simulink model "Quadrotor_Controller"  (R2018b)
settings: Solver=ode14x  StartTime=0.0  StopTime=10  FixedStep=1/100  RelTol=1e-3  EnableMultiTasking=on
undefined symbols (not defined in the file): Ap, cd, DiscIntNeverNeededParam, kt, L, Newton, Pitch_0, Raphson, rho, Roll_0, Rp, X, Y, Z
libraries: sm_lib x122, fl_lib x69, nesl_utility x14, sharedtransform x12, simulink x5, Electrical_Library x4, Mechanical_Library x4
(part 1 of 4)
settings Model: Creator=ppreethi  LastModifiedBy=standard
settings SolverCC: ExtrapolationOrder=2
settings DataIOCC: LimitDataPoints=on  SaveFormat=Array  InspectSignalLogs=on
settings OptimizationCC: BlockReduction=off  DefaultParameterBehavior=Inlined  OptimizeBlockIOStorage=off  BufferReuse=off  GlobalBufferReuse=off  ExpressionFolding=off  LocalBlockOutputs=off  LifeSpan=inf  OptimizeDataStoreBuffers=off  BusAssignmentInplaceUpdate=off
settings DebuggingCC: UnderspecifiedInitializationDetection=Classic  MergeDetectMultiDrivingBlocksExec=none  SolverPrmCheckMsg=warning  ParameterPrecisionLossMsg=none  BusObjectLabelMismatch=error  StateNameClashWarn=warning  StrictBusMsg=ErrorOnBusTreatedAsVector  NonBusSignalsTreatedAsBus=warning  SFUnexpectedBacktrackingDiag=warning  SFNoUnconditionalDefaultTransitionDiag=warning  SFExecutionAtInitializationDiag=none
settings HardwareCC: ProdBitPerPointer=32  ProdBitPerSizeT=32  ProdBitPerPtrDiffT=32  ProdLargestAtomicFloat=None  ProdWordSize=32  ProdHWDeviceType=Generic->32-bit x86 compatible
settings ModelReferenceCC: PropagateSignalLabelsOutOfModel=off
settings SFSimCC: SimUseLocalCustomCode=off
settings RTWCC: SystemTargetFile=xpctarget.tlc  TLCOptions=-axPCModelStackSizeKB=1024  TemplateMakefile=xpc_default_tmf  Description=xPC Target  RTWUseLocalCustomCode=off  RTWCompilerOptimization=on
settings CodeAppCC: StateflowObjectComments=on
settings TargetCC: CodeReplacementLibrary=XPC_BLAS  ParMdlRefBuildCompliant=on  ConcurrentExecutionCompliant=on  MatFileLogging=on  PreserveStateflowLocalDataDimensions=off  MATLABClassNameForMDSCustomization=xpcAperiodicCustomization
settings ConfigComp: CovMetricSettings=dw  CovHtmlReporting=on  CovSaveCumulativeToWorkspaceVar=on  CovSaveSingleToWorkspaceVar=on  CovExternalEMLEnable=off  CovSFcnEnable=off
settings SimscapeCC: SimscapeNormalizeSystem=off
settings ConfigurationSet: Description=SimMechanics 2G
settings ExplorerConfigSet: InternalSimMechanicsExplorerSettings="<ExplorerConfiguration><canonicalview>default</canonicalview><AnimationSetting><BasePlaybackSpeed>1.0</BasePlaybackSpeed><PlaybackSpeedFactor>1.0</PlaybackSpeedFactor></AnimationSetting><TilePanel><TileInfo><Tiles Columns=\"1\" Count=\"1\" Rows=\"1\"><Column Left=\"2\" Weight=\"1\"/><Column Left=\"1669\"/><Row Top=\"2\" Weight=\"1\"/><Row Top=\"1032\"/><Tile Height=\"1\" Width=\"1\" X=\"0\" Y=\"0\"/></Tiles></TileInfo><SceneInfo><SceneViewer><BGColor><R>1</R><G>1</G><B>1</B></BGColor><Camera><Position><X>-0.98734234069472837</X><Y>-2.5766196877608176</Y><Z>-0.21434917441758128</Z></Position><Center><X>-0.36548137966941641</X><Y>0.086653013342029503</Y><Z>0.52407155472837563</Z></Center><Up><X>-0.18648657026384141</X><Y>0.30268994651916503</Y><Z>-0.93466654769893953</Z></Up><Left>-0.88113891027964153</Left><Right>0.88113891027964153</Right><Bottom>-0.94141860281001366</Bottom><Top>0.94141860281001366</Top></Camera></SceneViewer></SceneInfo></TilePanel></ExplorerConfiguration>"

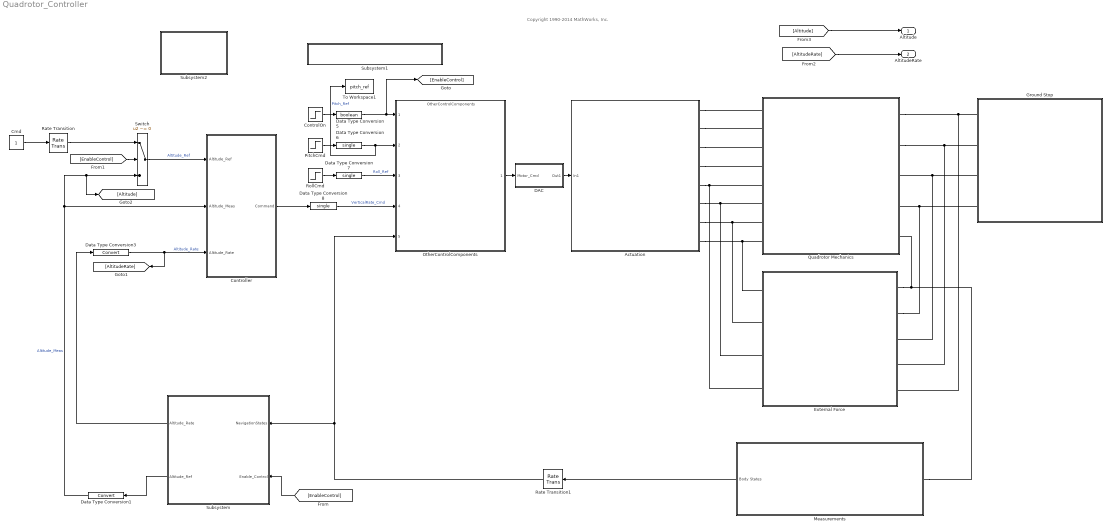
== system Quadrotor_Controller ==
  note: Copyright 1990-2014 MathWorks, Inc.
  Actuation : Subsystem
      mask Display: image('motor.png')
  Cmd : Constant
  ControlOn : Step  Time=5  SampleTime=0.01
  Controller : Subsystem  VariantControl=DesktopMode
  DAC : Subsystem
      mask Display: disp('DAC')
  Data Type Conversion1 : DataTypeConversion
  Data Type Conversion3 : DataTypeConversion
  Data Type Conversion5 : DataTypeConversion  OutDataTypeStr=boolean
  Data Type Conversion6 : DataTypeConversion  OutDataTypeStr=single
  Data Type Conversion7 : DataTypeConversion  OutDataTypeStr=single
  Data Type Conversion8 : DataTypeConversion  OutDataTypeStr=single
  External Force : Subsystem
      mask Display: image('rotor.png')
  Ground Stop : Subsystem  mask{Roll0=Roll_0, Pitch0=Pitch_0, Yaw0=0, Damp=0.7, Spring=1e2, Length=-0.083057999999999979068, GRoll=0, GPitch=0, Alt=1}
      mask prompts: Roll0 "Init Roll"; Pitch0 "Init Pitch"; Yaw0 "Init Yaw"; Damp "Damping"; Spring "Spring Constant"; Length "Distance from Center to Motor"; GRoll "Ground Roll"; GPitch "Ground Pitch"; Alt "Initial Altitude"
      mask init:
      | blk = gcb;
      | if Alt<0
      |     Alt = 0;
      |     set_param(blk,'Alt','0')
      |     warning('Cannot Initialize Below Zero Altitude');
      | end
      mask Display: image('earth.png')
  Measurements : Subsystem
  OtherControlComponents : ModelReference  ModelNameDialog=OtherControlComponents  SimulationMode=Normal  ModelReferenceVersion=1.148
  PitchCmd : Step  Time=8  After=0  SampleTime=0.01
  Quadrotor Mechanics : Subsystem
  Rate Transition : RateTransition  OutPortSampleTime=0.01
  Rate Transition1 : RateTransition
  RollCmd : Step  Time=8  After=0  SampleTime=0.01
  Subsystem : Subsystem
  Subsystem1 : Subsystem
      settings: OpenFcn=|
      | %%Set Variant to Real-time
      | HIL=1;
      | Desktop=0;
      | set_param(gcs,'SimulationMode','external');
      mask Display: disp('Real-time Settings')
  Subsystem2 : Subsystem
      settings: OpenFcn=|
      | %%Set Variant to Real-time
      | HIL=0;
      | Desktop=1;
      | set_param(gcs,'SimulationMode','normal');
      mask Display: disp('Desktop Settings')
  Switch : Switch  Criteria=u2 ~= 0
  To Workspace1 : ToWorkspace  VariableName=pitch_ref  SaveFormat=Timeseries  SampleTime=-1
  Altitude : Outport
  AltitudeRate : Outport  Port=2
  wires:
  Measurements/1(Body States) -> Rate Transition1/1
  PitchCmd/1 -> Data Type Conversion6/1
  RollCmd/1 -> Data Type Conversion7/1
  Rate Transition1/1 -> Subsystem/1(NavigationStates), OtherControlComponents/5
  Subsystem/2(Altitude_Ref) -> Data Type Conversion1/1
  Controller/1(Command) -> Data Type Conversion8/1
  Data Type Conversion1/1 -> Controller/2(Altitude_Meas), Switch/3, [Altitude]  "Altitude_Meas"
  Switch/1 -> Controller/1(Altitude_Ref)  "Altitude_Ref"
  ControlOn/1 -> Data Type Conversion5/1
  Cmd/1 -> Rate Transition/1
  Rate Transition/1 -> Switch/1
  Subsystem/1(Altitude_Rate) -> Data Type Conversion3/1
  Data Type Conversion3/1 -> [AltitudeRate], Controller/3(Altitude_Rate)  "Altitude_Rate"
  [EnableControl] -> Subsystem/2(Enable_Control)
  [EnableControl] -> Switch/2
  Data Type Conversion5/1 -> [EnableControl], OtherControlComponents/1
  Data Type Conversion6/1 -> To Workspace1/1, OtherControlComponents/2  "Pitch_Ref"
  Data Type Conversion7/1 -> OtherControlComponents/3  "Roll_Ref"
  Data Type Conversion8/1 -> OtherControlComponents/4  "VerticalRate_Cmd"
  OtherControlComponents/1 -> DAC/1(Motor_Cmd)
  DAC/1(Out1) -> Actuation/1(In1)
  [Altitude] -> Altitude/1
  [AltitudeRate] -> AltitudeRate/1
  connections:
  Quadrotor Mechanics/LConn8 -- External Force/LConn1 -- Actuation/RConn8
  External Force/LConn2 -- Actuation/RConn7 -- Quadrotor Mechanics/LConn7
  External Force/LConn4 -- Quadrotor Mechanics/LConn5 -- Actuation/RConn5
  Ground Stop/RConn1 -- Quadrotor Mechanics/RConn1 -- External Force/RConn5
  Ground Stop/RConn3 -- External Force/RConn3 -- Quadrotor Mechanics/RConn3
  Ground Stop/RConn2 -- Quadrotor Mechanics/RConn2 -- External Force/RConn4
  Ground Stop/RConn4 -- External Force/RConn2 -- Quadrotor Mechanics/RConn4
  Actuation/RConn4 -- Quadrotor Mechanics/LConn4
  Actuation/RConn3 -- Quadrotor Mechanics/LConn3
  Actuation/RConn2 -- Quadrotor Mechanics/LConn2
  External Force/RConn1 -- Quadrotor Mechanics/RConn5 -- Measurements/LConn1
  Actuation/RConn1 -- Quadrotor Mechanics/LConn1
  Quadrotor Mechanics/LConn6 -- Actuation/RConn6 -- External Force/LConn3

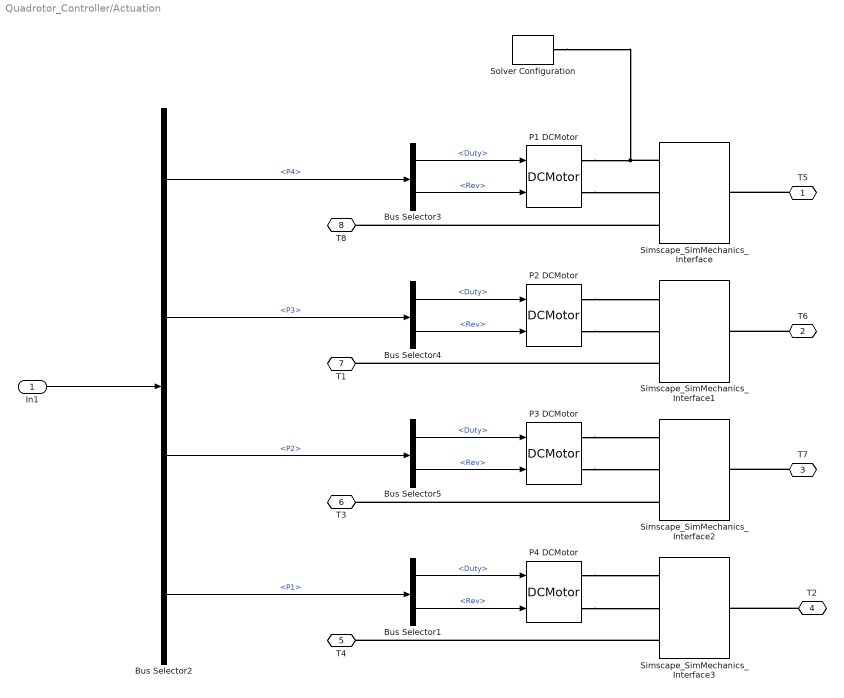
== system Quadrotor_Controller/Actuation ==
  In1 : Inport  OutDataTypeStr=Bus: MotorCommands
  " P1 DCMotor" : Electrical_Library/ DCMotor  SystemSampleTime=-1
  " P2 DCMotor" : Electrical_Library/ DCMotor  SystemSampleTime=-1
  " P3 DCMotor" : Electrical_Library/ DCMotor  SystemSampleTime=-1
  " P4 DCMotor" : Electrical_Library/ DCMotor  SystemSampleTime=-1
  Bus Selector{1,3..5} (4 alike) : BusSelector  OutputSignals=Duty,Rev
  Bus Selector2 : BusSelector  OutputSignals=P4,P3,P2,P1
  Simscape_SimMechanics_Interface{,1..3} (4 alike) : Mechanical_Library/Simscape_SimMechanics_Interface  SystemSampleTime=-1
  Solver Configuration : nesl_utility/Solver Configuration  PhysicalDomain=network_engine_domain  SubClassName=solver  LeftPortType=input  RightPortType=generic  Tones=[]  Harmonics=[]  SimulateNoise=off  Profile=off  UseLocalSampling=off  EnableSwitchedLinearOptims=on  FrequencyDomain=off  UseCCode=off  RelTol=0.001  AbsTol=1e-06  MinStep=1e-09  ToWorkspace=off  RevertToSquareIcSolve=off  NumHomotopyIterations=100  PhasorMode=off  PhasorModeNumHarmonics=1  DoDC=off  ResidualTolerance=1e-09  UseLocalSolver=off  LocalSolverChoice=NE_BACKWARD_EULER_ADVANCER  LocalSolverSampleTime=0.001  DoFixedCost=off  MaxNonlinIter=3  MaxModeIter=2  LinearAlgebra=Sparse  EquationFormulation=NE_TIME_EF  DelaysMemoryBudget=1024  AutomaticFiltering=on  FilteringTimeConstant=0.001  PartitionStorageMethod=AS_NEEDED  PartitionMemoryBudget=1024
  T5 : PMIOPort  Side=Right
  T6 : PMIOPort  Port=2  Side=Right
  T7 : PMIOPort  Port=3  Side=Right
  T2 : PMIOPort  Port=4  Side=Right
  T4 : PMIOPort  Port=5  Side=Right
  T3 : PMIOPort  Port=6  Side=Right
  T1 : PMIOPort  Port=7  Side=Right
  T8 : PMIOPort  Port=8  Side=Right
  wires:
  Bus Selector3/2 -> " P1 DCMotor"/2  "<Rev>"
  Bus Selector3/1 -> " P1 DCMotor"/1  "<Duty>"
  Bus Selector2/1 -> Bus Selector3/1  "<P4>"
  Bus Selector2/4 -> Bus Selector1/1  "<P1>"
  Bus Selector2/2 -> Bus Selector4/1  "<P3>"
  Bus Selector4/2 -> " P2 DCMotor"/2  "<Rev>"
  Bus Selector4/1 -> " P2 DCMotor"/1  "<Duty>"
  Bus Selector5/2 -> " P3 DCMotor"/2  "<Rev>"
  Bus Selector5/1 -> " P3 DCMotor"/1  "<Duty>"
  Bus Selector1/2 -> " P4 DCMotor"/2  "<Rev>"
  Bus Selector1/1 -> " P4 DCMotor"/1  "<Duty>"
  In1/1 -> Bus Selector2/1
  Bus Selector2/3 -> Bus Selector5/1  "<P2>"
  connections:
  Simscape_SimMechanics_Interface/LConn1 -- " P1 DCMotor"/RConn1 -- Solver Configuration/RConn1
  " P1 DCMotor"/RConn2 -- Simscape_SimMechanics_Interface/LConn2
  " P2 DCMotor"/RConn2 -- Simscape_SimMechanics_Interface1/LConn2
  " P2 DCMotor"/RConn1 -- Simscape_SimMechanics_Interface1/LConn1
  " P3 DCMotor"/RConn2 -- Simscape_SimMechanics_Interface2/LConn2
  " P3 DCMotor"/RConn1 -- Simscape_SimMechanics_Interface2/LConn1
  " P4 DCMotor"/RConn1 -- Simscape_SimMechanics_Interface3/LConn1
  " P4 DCMotor"/RConn2 -- Simscape_SimMechanics_Interface3/LConn2
  T5/RConn1 -- Simscape_SimMechanics_Interface/RConn1
  T6/RConn1 -- Simscape_SimMechanics_Interface1/RConn1
  T7/RConn1 -- Simscape_SimMechanics_Interface2/RConn1
  T2/RConn1 -- Simscape_SimMechanics_Interface3/RConn1
  Simscape_SimMechanics_Interface3/LConn3 -- T4/RConn1
  Simscape_SimMechanics_Interface2/LConn3 -- T3/RConn1
  Simscape_SimMechanics_Interface1/LConn3 -- T1/RConn1
  Simscape_SimMechanics_Interface/LConn3 -- T8/RConn1

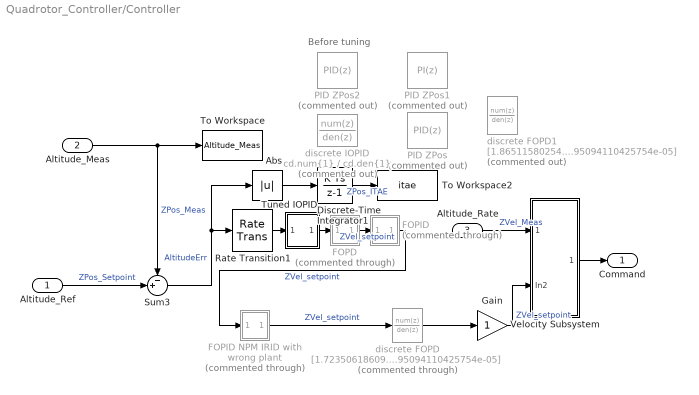
== system Quadrotor_Controller/Controller ==
  note: Before tuning
  Altitude_Ref : Inport
  Altitude_Meas : Inport  Port=2
  Altitude_Rate : Inport  Port=3
  Abs : Abs
  Discrete-Time Integrator1 : DiscreteIntegrator  SampleTime=-1  ICPrevOutput=DiscIntNeverNeededParam  ICPrevScaledInput=DiscIntNeverNeededParam
  FOPD : Subsystem  Commented=through
  FOPID : Subsystem  Commented=through
  FOPID NPM IRID with wrong plant : Subsystem  Commented=through
  Gain : Gain
  PID ZPos : simulink/Continuous/PID Controller  Commented=on  Controller=PID  Form=Parallel  TimeDomain=Discrete-time  SampleTime=0.01  IntegratorMethod=Forward Euler  FilterMethod=Forward Euler  ControllerParametersSource=internal  P=-0.572143949283884  I=-0.0379651986984248  D=-2.15558399471208  UseFilter=off  N=156.048759102889  TunerSelectOption=Transfer Function Based (PID Tuner App)  InitialConditionSource=internal  InitialConditionForIntegrator=0  InitialConditionForFilter=0  DifferentiatorICPrevScaledInput=0  ExternalReset=none  TrackingMode=off  Kt=1  LimitOutput=on  UpperSaturationLimit=10  LowerSaturationLimit=-10  LinearizeAsGain=on  AntiWindupMode=back-calculation  Kb=1  POutMin=[]  POutMax=[]  IOutMin=[]  IOutMax=[]  DOutMin=[]  DOutMax=[]  NOutMin=[]  NOutMax=[]  SumOutMin=[]  SumOutMax=[]  SaturationOutMin=[]  SaturationOutMax=[]  PParamMin=[]  PParamMax=[]  IParamMin=[]  IParamMax=[]  DParamMin=[]  DParamMax=[]  NParamMin=[]  NParamMax=[]  KbParamMin=[]  KbParamMax=[]  KtParamMin=[]  KtParamMax=[]  KbOutMin=[]  KbOutMax=[]  KtOutMin=[]  KtOutMax=[]  IntegratorOutMin=[]  IntegratorOutMax=[]  FilterOutMin=[]  FilterOutMax=[]  SumI1OutMin=[]  SumI1OutMax=[]  SumI2OutMin=[]  SumI2OutMax=[]  SumI3OutMin=[]  SumI3OutMax=[]  SumI4OutMin=[]  SumI4OutMax=[]  SumDOutMin=[]  SumDOutMax=[]  DifferentiatorOutMin=[]  DifferentiatorOutMax=[]  FilterDiffOutCoefMin=[]  FilterDiffOutCoefMax=[]  ReciprocalOutMin=[]  ReciprocalOutMax=[]  SumDenOutMin=[]  SumDenOutMax=[]  SumNumOutMin=[]  SumNumOutMax=[]  DivideOutMin=[]  DivideOutMax=[]  IntegratorContinuousStateAttributes=''  IntegratorStateMustResolveToSignalObject=off  IntegratorRTWStateStorageClass=Auto  FilterContinuousStateAttributes=''  FilterStateMustResolveToSignalObject=off  FilterRTWStateStorageClass=Auto  ParallelPVariant=InternalParameters  IdealPVariant=Disabled  IVariant=InternalParameters  DVariant=InternalParameters  IntegratorVariant=Discrete  SatVariant=Enabled  AWVariant=BackCalculation  PCopyVariant=Disabled  TRVariant=Disabled  FdbkBlocksVariant=Forward  IdealPFdbkVariant=Disabled  SatFdbkVariant=Disabled  DerivativeFilterVariant=Differentiator  NVariant=Passthrough  NCopyVariant=Disabled_SignalSpec  FilterICVariant=InternalICsDifferentiator  IntegratorICVariant=InternalICs  ExternalResetVariant=Disabled  TRSumVariant=Passthrough  SumFdbkVariant=Disabled  SumVariant=Sum_PID
  PID ZPos1 : simulink/Continuous/PID Controller  Commented=on  Controller=PI  Form=Parallel  TimeDomain=Discrete-time  SampleTime=0.01  IntegratorMethod=Forward Euler  FilterMethod=Forward Euler  ControllerParametersSource=internal  P=3.31239291008358  I=4.5948345994664  D=-0.0090752929990825  UseFilter=on  N=156.048759102889  TunerSelectOption=Transfer Function Based (PID Tuner App)  InitialConditionSource=internal  InitialConditionForIntegrator=0  InitialConditionForFilter=0  DifferentiatorICPrevScaledInput=0  ExternalReset=none  TrackingMode=off  Kt=1  LimitOutput=on  UpperSaturationLimit=10  LowerSaturationLimit=-10  LinearizeAsGain=on  AntiWindupMode=back-calculation  Kb=1  POutMin=[]  POutMax=[]  IOutMin=[]  IOutMax=[]  DOutMin=[]  DOutMax=[]  NOutMin=[]  NOutMax=[]  SumOutMin=[]  SumOutMax=[]  SaturationOutMin=[]  SaturationOutMax=[]  PParamMin=[]  PParamMax=[]  IParamMin=[]  IParamMax=[]  DParamMin=[]  DParamMax=[]  NParamMin=[]  NParamMax=[]  KbParamMin=[]  KbParamMax=[]  KtParamMin=[]  KtParamMax=[]  KbOutMin=[]  KbOutMax=[]  KtOutMin=[]  KtOutMax=[]  IntegratorOutMin=[]  IntegratorOutMax=[]  FilterOutMin=[]  FilterOutMax=[]  SumI1OutMin=[]  SumI1OutMax=[]  SumI2OutMin=[]  SumI2OutMax=[]  SumI3OutMin=[]  SumI3OutMax=[]  SumI4OutMin=[]  SumI4OutMax=[]  SumDOutMin=[]  SumDOutMax=[]  DifferentiatorOutMin=[]  DifferentiatorOutMax=[]  FilterDiffOutCoefMin=[]  FilterDiffOutCoefMax=[]  ReciprocalOutMin=[]  ReciprocalOutMax=[]  SumDenOutMin=[]  SumDenOutMax=[]  SumNumOutMin=[]  SumNumOutMax=[]  DivideOutMin=[]  DivideOutMax=[]  IntegratorContinuousStateAttributes=''  IntegratorStateMustResolveToSignalObject=off  IntegratorRTWStateStorageClass=Auto  FilterContinuousStateAttributes=''  FilterStateMustResolveToSignalObject=off  FilterRTWStateStorageClass=Auto  ParallelPVariant=InternalParameters  IdealPVariant=Disabled  IVariant=InternalParameters  DVariant=Disabled  IntegratorVariant=Discrete  SatVariant=Enabled  AWVariant=BackCalculation  PCopyVariant=Disabled  TRVariant=Disabled  FdbkBlocksVariant=Forward  IdealPFdbkVariant=Disabled  SatFdbkVariant=Disabled  DerivativeFilterVariant=Disabled  NVariant=Disabled  NCopyVariant=Disabled_SignalSpec  FilterICVariant=Disabled  IntegratorICVariant=InternalICs  ExternalResetVariant=Disabled  TRSumVariant=Passthrough  SumFdbkVariant=Disabled  SumVariant=Sum_PI
  PID ZPos2 : simulink/Continuous/PID Controller  Commented=on  Controller=PID  Form=Parallel  TimeDomain=Discrete-time  SampleTime=0.01  IntegratorMethod=Forward Euler  FilterMethod=Forward Euler  ControllerParametersSource=internal  P=3.2  I=2  D=0  UseFilter=off  N=156.048759102889  TunerSelectOption=Transfer Function Based (PID Tuner App)  InitialConditionSource=internal  InitialConditionForIntegrator=0  InitialConditionForFilter=0  DifferentiatorICPrevScaledInput=0  ExternalReset=none  TrackingMode=off  Kt=1  LimitOutput=on  UpperSaturationLimit=10  LowerSaturationLimit=-10  LinearizeAsGain=on  AntiWindupMode=back-calculation  Kb=1  POutMin=[]  POutMax=[]  IOutMin=[]  IOutMax=[]  DOutMin=[]  DOutMax=[]  NOutMin=[]  NOutMax=[]  SumOutMin=[]  SumOutMax=[]  SaturationOutMin=[]  SaturationOutMax=[]  PParamMin=[]  PParamMax=[]  IParamMin=[]  IParamMax=[]  DParamMin=[]  DParamMax=[]  NParamMin=[]  NParamMax=[]  KbParamMin=[]  KbParamMax=[]  KtParamMin=[]  KtParamMax=[]  KbOutMin=[]  KbOutMax=[]  KtOutMin=[]  KtOutMax=[]  IntegratorOutMin=[]  IntegratorOutMax=[]  FilterOutMin=[]  FilterOutMax=[]  SumI1OutMin=[]  SumI1OutMax=[]  SumI2OutMin=[]  SumI2OutMax=[]  SumI3OutMin=[]  SumI3OutMax=[]  SumI4OutMin=[]  SumI4OutMax=[]  SumDOutMin=[]  SumDOutMax=[]  DifferentiatorOutMin=[]  DifferentiatorOutMax=[]  FilterDiffOutCoefMin=[]  FilterDiffOutCoefMax=[]  ReciprocalOutMin=[]  ReciprocalOutMax=[]  SumDenOutMin=[]  SumDenOutMax=[]  SumNumOutMin=[]  SumNumOutMax=[]  DivideOutMin=[]  DivideOutMax=[]  IntegratorContinuousStateAttributes=''  IntegratorStateMustResolveToSignalObject=off  IntegratorRTWStateStorageClass=Auto  FilterContinuousStateAttributes=''  FilterStateMustResolveToSignalObject=off  FilterRTWStateStorageClass=Auto  ParallelPVariant=InternalParameters  IdealPVariant=Disabled  IVariant=InternalParameters  DVariant=InternalParameters  IntegratorVariant=Discrete  SatVariant=Enabled  AWVariant=BackCalculation  PCopyVariant=Disabled  TRVariant=Disabled  FdbkBlocksVariant=Forward  IdealPFdbkVariant=Disabled  SatFdbkVariant=Disabled  DerivativeFilterVariant=Differentiator  NVariant=Passthrough  NCopyVariant=Disabled_SignalSpec  FilterICVariant=InternalICsDifferentiator  IntegratorICVariant=InternalICs  ExternalResetVariant=Disabled  TRSumVariant=Passthrough  SumFdbkVariant=Disabled  SumVariant=Sum_PID
  Rate Transition1 : RateTransition  OutPortSampleTime=0.01
  Sum3 : Sum  Inputs=-+|
  To Workspace : ToWorkspace  VariableName=Altitude_Meas  SaveFormat=Timeseries  SampleTime=-1
  To Workspace2 : ToWorkspace  VariableName=itae  SaveFormat=Timeseries  SampleTime=-1
  Tuned IOPID : Subsystem
  Velocity Subsystem : Subsystem
  discrete FOPD : DiscreteTransferFcn  Commented=through  Numerator=[1.72350618609064,-5.70339892298403,7.11891293410561,-4.08227197470563,1.02223847578118,-0.0786444191365231]  Denominator=[0.0101201839324044,-0.0228427827690589,0.0162967440497079,-0.00320636053105791,-0.000423005899049262,8.95094110425754e-05]  SampleTime=0.01
  discrete FOPD1 : DiscreteTransferFcn  Commented=on  Numerator=[1.86511580254824,-6.20360416522752,7.77951053722034,-4.47930158754086,1.12529607747831,-0.0867420445559554]  Denominator=[0.0101201839324044,-0.0228427827690589,0.0162967440497079,-0.00320636053105791,-0.000423005899049262,8.95094110425754e-05]  SampleTime=0.01
  discrete IOPID : DiscreteTransferFcn  Description=This one makes saturation, because no anti-windup  Commented=on  Numerator=cd.num{1}  Denominator=cd.den{1}  SampleTime=0.01
  Command : Outport
  wires:
  Altitude_Ref/1 -> Sum3/2  "ZPos_Setpoint"
  Altitude_Meas/1 -> To Workspace/1, Sum3/1  "ZPos_Meas"
  discrete FOPD/1 -> Gain/1
  Sum3/1 -> Abs/1, Rate Transition1/1  "AltitudeErr"
  Discrete-Time Integrator1/1 -> To Workspace2/1  "ZPos_ITAE"
  Abs/1 -> Discrete-Time Integrator1/1
  Tuned IOPID/1(Out1) -> FOPD/1(In1)
  Rate Transition1/1 -> Tuned IOPID/1(In1)
  Altitude_Rate/1 -> Velocity Subsystem/1(Altitude_Rate)  "ZVel_Meas"
  Gain/1 -> Velocity Subsystem/2(In2)  "ZVel_setpoint"
  Velocity Subsystem/1(Command) -> Command/1
  FOPD/1(Out1) -> FOPID/1(In1)  "ZVel_setpoint"
  FOPID/1(Out1) -> FOPID NPM IRID with wrong plant/1(In1)  "ZVel_setpoint"
  FOPID NPM IRID with wrong plant/1(Out1) -> discrete FOPD/1  "ZVel_setpoint"

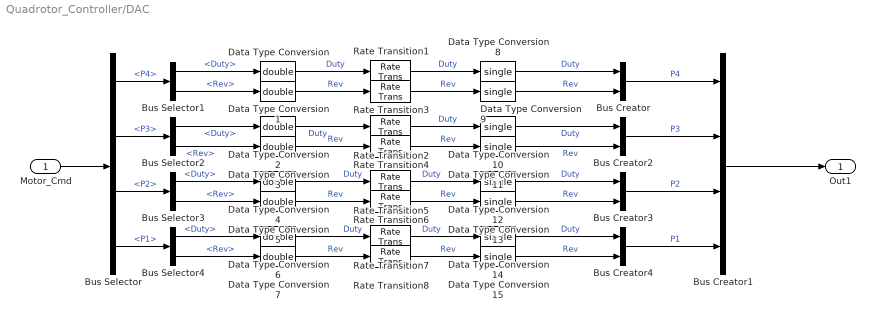
== system Quadrotor_Controller/DAC ==
  Motor_Cmd : Inport
  Bus Creator{,2..4} (4 alike) : BusCreator  Inputs='Duty','Rev'  OutDataTypeStr=Bus: PWMBus
  Bus Creator1 : BusCreator  Inputs='P4','P3','P2','P1'  OutDataTypeStr=Bus: MotorCommands
  Bus Selector : BusSelector  OutputSignals=P4,P3,P2,P1
  Bus Selector{1..4} (4 alike) : BusSelector  OutputSignals=Duty,Rev
  Data Type Conversion{,1..7} (8 alike) : DataTypeConversion  OutDataTypeStr=double
  Data Type Conversion{8..15} (8 alike) : DataTypeConversion  OutDataTypeStr=single
  Rate Transition{1..8} (8 alike) : RateTransition
  Out1 : Outport
  wires:
  Motor_Cmd/1 -> Bus Selector/1
  Bus Creator1/1 -> Out1/1
  Bus Selector/1 -> Bus Selector1/1  "<P4>"
  Bus Selector/2 -> Bus Selector2/1  "<P3>"
  Bus Selector/3 -> Bus Selector3/1  "<P2>"
  Bus Selector/4 -> Bus Selector4/1  "<P1>"
  Bus Selector1/1 -> Data Type Conversion/1  "<Duty>"
  Bus Selector1/2 -> Data Type Conversion1/1  "<Rev>"
  Data Type Conversion8/1 -> Bus Creator/1  "Duty"
  Data Type Conversion9/1 -> Bus Creator/2  "Rev"
  Bus Selector2/1 -> Data Type Conversion2/1  "<Duty>"
  Bus Selector2/2 -> Data Type Conversion3/1  "<Rev>"
  Bus Selector3/1 -> Data Type Conversion4/1  "<Duty>"
  Bus Selector3/2 -> Data Type Conversion5/1  "<Rev>"
  Bus Selector4/1 -> Data Type Conversion6/1  "<Duty>"
  Bus Selector4/2 -> Data Type Conversion7/1  "<Rev>"
  Bus Creator/1 -> Bus Creator1/1  "P4"
  Bus Creator3/1 -> Bus Creator1/3  "P2"
  Bus Creator2/1 -> Bus Creator1/2  "P3"
  Bus Creator4/1 -> Bus Creator1/4  "P1"
  Data Type Conversion1/1 -> Rate Transition3/1  "Rev"
  Data Type Conversion/1 -> Rate Transition1/1  "Duty"
  Data Type Conversion3/1 -> Rate Transition4/1  "Rev"
  Data Type Conversion2/1 -> Rate Transition2/1  "Duty"
  Data Type Conversion5/1 -> Rate Transition6/1  "Rev"
  Data Type Conversion4/1 -> Rate Transition5/1  "Duty"
  Data Type Conversion7/1 -> Rate Transition8/1  "Rev"
  Data Type Conversion6/1 -> Rate Transition7/1  "Duty"
  Rate Transition1/1 -> Data Type Conversion8/1  "Duty"
  Rate Transition3/1 -> Data Type Conversion9/1  "Rev"
  Data Type Conversion10/1 -> Bus Creator2/1  "Duty"
  Data Type Conversion11/1 -> Bus Creator2/2  "Rev"
  Rate Transition2/1 -> Data Type Conversion10/1  "Duty"
  Rate Transition4/1 -> Data Type Conversion11/1  "Rev"
  Data Type Conversion12/1 -> Bus Creator3/1  "Duty"
  Data Type Conversion13/1 -> Bus Creator3/2  "Rev"
  Rate Transition5/1 -> Data Type Conversion12/1  "Duty"
  Rate Transition6/1 -> Data Type Conversion13/1  "Rev"
  Data Type Conversion14/1 -> Bus Creator4/1  "Duty"
  Data Type Conversion15/1 -> Bus Creator4/2  "Rev"
  Rate Transition7/1 -> Data Type Conversion14/1  "Duty"
  Rate Transition8/1 -> Data Type Conversion15/1  "Rev"

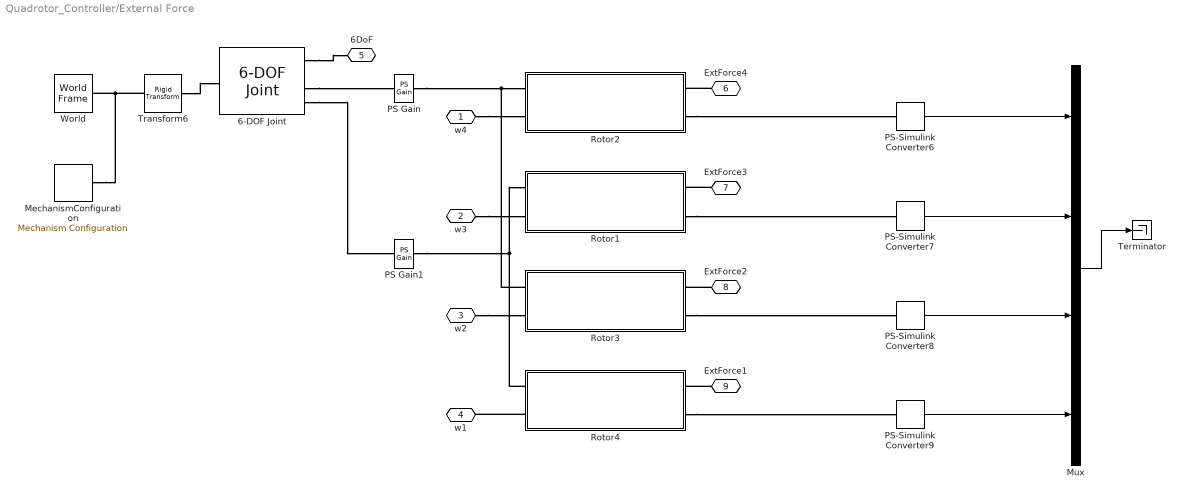
== system Quadrotor_Controller/External Force ==
  6-DOF Joint : sm_lib/Joints/6-DOF Joint  SenseConstraintForce=off  SenseConstraintForceX=off  SenseConstraintForceY=off  SenseConstraintForceZ=off  SenseConstraintTorque=off  SenseConstraintTorqueX=off  SenseConstraintTorqueY=off  SenseConstraintTorqueZ=off  SenseTotalForce=off  SenseTotalForceX=off  SenseTotalForceY=off  SenseTotalForceZ=off  SenseTotalTorque=off  SenseTotalTorqueX=off  SenseTotalTorqueY=off  SenseTotalTorqueZ=off  CompositeWrenchDir=FollowerOnBase  CompositeWrenchFrame=BaseFrame  PxEquilibriumPosition=0  PxEquilibriumPositionUnits=m  PxSpringStiffness=0  PxSpringStiffnessUnits=N/m  PxDampingCoefficient=0  PxDampingCoefficientUnits=N/(m/s)  PxTorqueActuationMode=NoTorque  PxMotionActuationMode=ComputedMotion  PxSensePosition=off  PxSenseVelocity=off  PxSenseAcceleration=off  PxSenseTorqueForce=off  PxPositionTargetSpecify=off  PxPositionTargetPriority=High  PxPositionTargetValue=0  PxPositionTargetValueUnits=m  PxVelocityTargetSpecify=off  PxVelocityTargetPriority=High  PxVelocityTargetValue=0  PxVelocityTargetValueUnits=m/s  PyEquilibriumPosition=0  PyEquilibriumPositionUnits=m  PySpringStiffness=0  PySpringStiffnessUnits=N/m  PyDampingCoefficient=0  PyDampingCoefficientUnits=N/(m/s)  PyTorqueActuationMode=NoTorque  PyMotionActuationMode=ComputedMotion  PySensePosition=off  PySenseVelocity=off  PySenseAcceleration=off  PySenseTorqueForce=off  PyPositionTargetSpecify=off  PyPositionTargetPriority=High  PyPositionTargetValue=0  PyPositionTargetValueUnits=m  PyVelocityTargetSpecify=off  PyVelocityTargetPriority=High  PyVelocityTargetValue=0  PyVelocityTargetValueUnits=m/s  PzEquilibriumPosition=0  PzEquilibriumPositionUnits=m  PzSpringStiffness=0  PzSpringStiffnessUnits=N/m  PzDampingCoefficient=0  PzDampingCoefficientUnits=N/(m/s)  PzTorqueActuationMode=NoTorque  PzMotionActuationMode=ComputedMotion  PzSensePosition=off  PzSenseVelocity=on  PzSenseAcceleration=off  PzSenseTorqueForce=off  PzPositionTargetSpecify=off  PzPositionTargetPriority=High  PzPositionTargetValue=-1  PzPositionTargetValueUnits=m  PzVelocityTargetSpecify=off  PzVelocityTargetPriority=High  PzVelocityTargetValue=0  PzVelocityTargetValueUnits=m/s  SphDefPosRotationMethod=None  SphDefPosRotationAngleUnits=deg  SphDefPosRotationStandardAxis=+Z  SphDefPosRotationAngle=0  SphDefPosRotationArbitraryAxis=[0 0 1]  SphDefPosFollAlignAxisA=+X  SphDefPosBaseAlignAxisA=+Y  SphDefPosFollAlignAxisB=+Y  SphDefPosBaseAlignAxisB=+Z  SphDefPosRotationSequenceAxes=FollowerAxes  SphDefPosRotationSequence=XYX  SphDefPosRotationSequenceAngles=[0 0 0]  SphDefPosRotationSequenceAnglesUnits=deg  SphDefPosRotationMatrix=[1 0 0; 0 1 0; 0 0 1]  SphEqPosRotationMethod=None  SphEqPosRotationAngleUnits=deg  SphEqPosRotationStandardAxis=+Z  SphEqPosRotationAngle=0  SphEqPosRotationArbitraryAxis=[0 0 1]  SphEqPosFollAlignAxisA=+X  SphEqPosBaseAlignAxisA=+Y  SphEqPosFollAlignAxisB=+Y  SphEqPosBaseAlignAxisB=+Z  SphEqPosRotationSequenceAxes=FollowerAxes  SphEqPosRotationSequence=XYX  SphEqPosRotationSequenceAngles=[0 0 0]  SphEqPosRotationSequenceAnglesUnits=deg  SphEqPosRotationMatrix=[1 0 0; 0 1 0; 0 0 1]  SphSpringStiffness=0  SphSpringStiffnessUnits=N*m/deg  SphDampingCoefficient=0  SphDampingCoefficientUnits=N*m/(deg/s)  SphActuateTorqueX=off  SphActuateTorqueY=off  SphActuateTorqueZ=off  SphActuateTorque=off  SphTorqueActuationMode=NoTorque  SphMotionActuationMode=ComputedMotion  SphActuationFrame=BaseFrame  SphSensePosition=off  SphSenseVelocityX=on  SphSenseVelocityY=on  SphSenseVelocityZ=off  SphSenseVelocity=off  SphSenseAccelerationX=off  SphSenseAccelerationY=off  SphSenseAccelerationZ=off  SphSenseAcceleration=off  SphSenseTorqueX=off  SphSenseTorqueY=off  SphSenseTorqueZ=off  SphSenseTorqueForce=off  SphSensingFrame=BaseFrame  SphPositionTargetRotationMethod=None  SphPositionTargetRotationAngleUnits=deg  SphPositionTargetRotationStandardAxis=+Z  SphPositionTargetRotationAngle=0  SphPositionTargetRotationArbitraryAxis=[0 0 1]  SphPositionTargetFollAlignAxisA=+X  SphPositionTargetBaseAlignAxisA=+Y  SphPositionTargetFollAlignAxisB=+Y  SphPositionTargetBaseAlignAxisB=+Z  SphPositionTargetRotationSequenceAxes=FollowerAxes  SphPositionTargetRotationSequence=XYX  SphPositionTargetRotationSequenceAngles=[0 0 0]  SphPositionTargetRotationSequenceAnglesUnits=deg  SphPositionTargetRotationMatrix=[1 0 0; 0 1 0; 0 0 1]  SphPositionTargetSpecify=off  SphPositionTargetPriority=High  SphVelocityTargetValue=[0 0 0]  SphVelocityTargetValueUnits=deg/s  SphVelocityTargetSpecify=off  SphVelocityTargetPriority=High  SphVelocityTargetInFollowerFrame=on
  MechanismConfiguration : sm_lib/Utilities/Mechanism Configuration  UniformGravity=Constant  GravityVector=[0 0 9.81]  GravityUnits=m/s^2  LinearizationDelta=0.001
  Mux : Mux
  PS Gain : fl_lib/Physical Signals/Functions/PS Gain  gain=pi/180
  PS Gain1 : fl_lib/Physical Signals/Functions/PS Gain  gain=pi/180
  PS-Simulink Converter{6..9} (4 alike) : nesl_utility/PS-Simulink Converter  PhysicalDomain=network_engine_domain  SubClassName=ps_output  LeftPortType=input  RightPortType=output  PseudoPeriodic=off  Frequencies=[]  Unit=1  AffineConversion=off
  Rotor1 : Subsystem
  Rotor2 : Subsystem
  Rotor3 : Subsystem
  Rotor4 : Subsystem
  Terminator : Terminator
  Transform6 : sm_lib/Frames and Transforms/Rigid Transform  TranslationMethod=None  TranslationStandardOffset=0  TranslationLengthUnit=m  TranslationStandardAxis=+Z  TranslationCartesianOffset=[0 0 0]  TranslationROffset=0  TranslationROffsetUnits=m  TranslationZOffset=0  TranslationZOffsetUnits=m  TranslationThetaOffset=0  TranslationThetaOffsetUnits=deg  RotationMethod=StandardAxis  RotationAngleUnits=deg  RotationStandardAxis=+X  RotationAngle=180  RotationArbitraryAxis=[0 0 1]  FollAlignAxisA=+X  BaseAlignAxisA=+Y  FollAlignAxisB=+Y  BaseAlignAxisB=+Z  RotationSequenceAxes=FollowerAxes  RotationSequence=XYX  RotationSequenceAngles=[0 0 0]  RotationSequenceAnglesUnits=deg  RotationMatrix=[1 0 0; 0 1 0; 0 0 1]
  World : sm_lib/Frames and Transforms/World Frame
  w4 : PMIOPort  Side=Left
  w3 : PMIOPort  Port=2  Side=Left
  w2 : PMIOPort  Port=3  Side=Left
  w1 : PMIOPort  Port=4  Side=Left
  6DoF : PMIOPort  Port=5  Side=Right
  ExtForce4 : PMIOPort  Port=6  Side=Right
  ExtForce3 : PMIOPort  Port=7  Side=Right
  ExtForce2 : PMIOPort  Port=8  Side=Right
  ExtForce1 : PMIOPort  Port=9  Side=Right
  wires:
  PS-Simulink Converter9/1 -> Mux/4
  PS-Simulink Converter8/1 -> Mux/3
  PS-Simulink Converter7/1 -> Mux/2
  PS-Simulink Converter6/1 -> Mux/1
  Mux/1 -> Terminator/1
  connections:
  ExtForce1/RConn1 -- Rotor4/RConn1
  Rotor4/RConn2 -- PS-Simulink Converter9/LConn1
  Rotor3/RConn2 -- PS-Simulink Converter8/LConn1
  w3/RConn1 -- Rotor1/LConn2
  Rotor1/RConn2 -- PS-Simulink Converter7/LConn1
  Rotor4/LConn1 -- Rotor1/LConn1 -- PS Gain1/RConn1
  ExtForce2/RConn1 -- Rotor3/RConn1
  Rotor3/LConn1 -- Rotor2/LConn1 -- PS Gain/RConn1
  Rotor2/RConn2 -- PS-Simulink Converter6/LConn1
  ExtForce3/RConn1 -- Rotor1/RConn1
  ExtForce4/RConn1 -- Rotor2/RConn1
  w4/RConn1 -- Rotor2/LConn2
  w2/RConn1 -- Rotor3/LConn2
  Rotor4/LConn2 -- w1/RConn1
  6-DOF Joint/RConn1 -- 6DoF/RConn1
  Transform6/RConn1 -- 6-DOF Joint/LConn1
  Transform6/LConn1 -- World/RConn1 -- MechanismConfiguration/RConn1
  6-DOF Joint/RConn4 -- PS Gain1/LConn1
  6-DOF Joint/RConn3 -- PS Gain/LConn1

== system Quadrotor_Controller/Ground Stop ==
  FloorStop1 : Subsystem
  FloorStop2 : Subsystem
  FloorStop3 : Subsystem
  FloorStop4 : Subsystem
  Ground : sm_lib/Body Elements/Solid  InertiaType=CalculateFromGeometry  Mass=1  MassUnits=kg  CenterOfMass=[0 0 0]  CenterOfMassUnits=m  MomentsOfInertia=[1 1 1]  MomentsOfInertiaUnits=kg*m^2  ProductsOfInertia=[0 0 0]  ProductsOfInertiaUnits=kg*m^2  BasedOnType=Density  Density=2000  DensityUnits=kg/(m^3)  DoExposeReferenceFrame=on  SerializedFrames=<Frames/>  GraphicType=FromGeometry  MarkerShape=Sphere  MarkerSize=10  MarkerSizeUnits=m  GraphicVisPropType=SimpleVisualProperties  GraphicDiffuseColor=[0.0 0.0 0.2]  GraphicSpecularColor=[0.5 0.5 0.5 1.0]  GraphicAmbientColor=[0.15 0.15 0.15 1.0]  GraphicEmissiveColor=[0.0 0.0 0.0 1.0]  GraphicShininess=75  GraphicOpacity=1.0  GeometryShape=Brick  RectangleSize=[1 1]  RectangleSizeUnits=m  BrickDimensions=[1 1 0.01]  BrickDimensionUnits=m  CylinderRadius=1  CylinderRadiusUnits=m  CylinderLength=1  CylinderLengthUnits=m  SphereRadius=1  SphereRadiusUnits=m  EllipsoidRadii=[1 1 1]  EllipsoidRadiiUnits=m  ExtrusionCrossSection=[1 1; -1 1; -1 -1; 1 -1]  ExtrusionCrossSectionUnits=m  ExtrusionLength=1  ExtrusionLengthUnits=m  PolygonNumSides=3  PolygonOuterRadius=1  PolygonOuterRadiusUnits=m  ExtGeomFileType=STL  ExtGeomFileUnits=m  RevolutionCrossSection=[1 1; 1 -1; 2 -1; 2 1]  RevolutionCrossSectionUnits=m  RevolutionExtent=Full  RevolutionAngle=180  RevolutionAngleUnits=deg
  Transform1 : sm_lib/Frames and Transforms/Rigid Transform  TranslationMethod=Cartesian  TranslationStandardOffset=0  TranslationLengthUnit=m  TranslationStandardAxis=+Z  TranslationCartesianOffset=[0 0 -Alt-0.038]  TranslationROffset=0  TranslationROffsetUnits=m  TranslationZOffset=0  TranslationZOffsetUnits=m  TranslationThetaOffset=0  TranslationThetaOffsetUnits=deg  RotationMethod=StandardAxis  RotationAngleUnits=deg  RotationStandardAxis=+X  RotationAngle=180  RotationArbitraryAxis=[0 0 1]  FollAlignAxisA=+X  BaseAlignAxisA=+Y  FollAlignAxisB=+Y  BaseAlignAxisB=+Z  RotationSequenceAxes=FollowerAxes  RotationSequence=XYX  RotationSequenceAngles=[0 0 0]  RotationSequenceAnglesUnits=deg  RotationMatrix=[1 0 0; 0 1 0; 0 0 1]
  Transform6 : sm_lib/Frames and Transforms/Rigid Transform  TranslationMethod=None  TranslationStandardOffset=0  TranslationLengthUnit=m  TranslationStandardAxis=+Z  TranslationCartesianOffset=[0 0 0]  TranslationROffset=0  TranslationROffsetUnits=m  TranslationZOffset=0  TranslationZOffsetUnits=m  TranslationThetaOffset=0  TranslationThetaOffsetUnits=deg  RotationMethod=StandardAxis  RotationAngleUnits=deg  RotationStandardAxis=+X  RotationAngle=180  RotationArbitraryAxis=[0 0 1]  FollAlignAxisA=+X  BaseAlignAxisA=+Y  FollAlignAxisB=+Y  BaseAlignAxisB=+Z  RotationSequenceAxes=FollowerAxes  RotationSequence=XYX  RotationSequenceAngles=[0 0 0]  RotationSequenceAnglesUnits=deg  RotationMatrix=[1 0 0; 0 1 0; 0 0 1]
  World1 : sm_lib/Frames and Transforms/World Frame
  Conn1 : PMIOPort  Side=Right
  Conn2 : PMIOPort  Port=2  Side=Right
  Conn3 : PMIOPort  Port=3  Side=Right
  Conn4 : PMIOPort  Port=4  Side=Right
  connections:
  FloorStop4/RConn1 -- Conn1/RConn1
  Conn3/RConn1 -- FloorStop1/RConn1
  Conn2/RConn1 -- FloorStop2/RConn1
  Conn4/RConn1 -- FloorStop3/RConn1
  FloorStop3/LConn1 -- Transform1/RConn1 -- Transform6/RConn1 -- FloorStop2/LConn1 -- FloorStop4/LConn1 -- FloorStop1/LConn1
  Transform6/LConn1 -- World1/RConn1
  Ground/RConn1 -- Transform1/LConn1

== system Quadrotor_Controller/Measurements ==
  Bus Mapping : Subsystem
  Subsystem : Subsystem
  "6dof " : PMIOPort  Side=Left
  Body States : Outport  OutDataTypeStr=Bus: NavigationStates
  wires:
  Bus Mapping/1(State) -> Body States/1  "BodyState"
  Subsystem/1(DCMbe) -> Bus Mapping/1(Attitude)
  Subsystem/4(OmegaZ) -> Bus Mapping/4(OmegaZ)  "Pos"
  Subsystem/2(OmegaX) -> Bus Mapping/2(OmegaX)  "Omega"
  Subsystem/5(ZPos) -> Bus Mapping/5(Position)  "Vel"
  Subsystem/3(OmegaY) -> Bus Mapping/3(OmegaY)
  Subsystem/6(ZVel) -> Bus Mapping/6(Velocity)
  connections:
  "6dof "/RConn1 -- Subsystem/LConn1

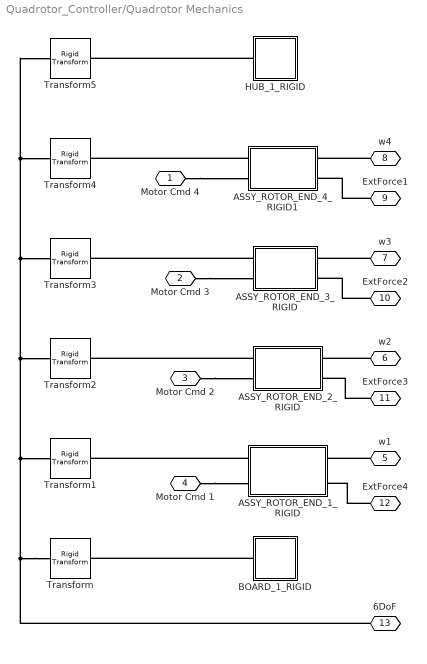
== system Quadrotor_Controller/Quadrotor Mechanics ==
  ASSY_ROTOR_END_1_RIGID : Subsystem
  ASSY_ROTOR_END_2_RIGID : Subsystem
  ASSY_ROTOR_END_3_RIGID : Subsystem
  ASSY_ROTOR_END_4_RIGID1 : Subsystem
  BOARD_1_RIGID : Subsystem
  HUB_1_RIGID : Subsystem
  Transform : sm_lib/Frames and Transforms/Rigid Transform  TranslationMethod=Cartesian  TranslationStandardOffset=0  TranslationLengthUnit=in  TranslationStandardAxis=+Z  TranslationCartesianOffset=[0 0 0.27699999999999997]  TranslationROffset=0  TranslationROffsetUnits=m  TranslationZOffset=0  TranslationZOffsetUnits=m  TranslationThetaOffset=0  TranslationThetaOffsetUnits=deg  RotationMethod=ArbitraryAxis  RotationAngleUnits=rad  RotationStandardAxis=+Z  RotationAngle=2.3561943620144121  RotationArbitraryAxis=[-0 -0 -0.99999999999999989]  FollAlignAxisA=+X  BaseAlignAxisA=+Y  FollAlignAxisB=+Y  BaseAlignAxisB=+Z  RotationSequenceAxes=FollowerAxes  RotationSequence=XYX  RotationSequenceAngles=[0 0 0]  RotationSequenceAnglesUnits=deg  RotationMatrix=[1 0 0; 0 1 0; 0 0 1]
  Transform1 : sm_lib/Frames and Transforms/Rigid Transform  TranslationMethod=Cartesian  TranslationStandardOffset=0  TranslationLengthUnit=in  TranslationStandardAxis=+Z  TranslationCartesianOffset=[0.085999999999999979 -5.5118110236220464e-05 5.5118110236220464e-05]  TranslationROffset=0  TranslationROffsetUnits=m  TranslationZOffset=0  TranslationZOffsetUnits=m  TranslationThetaOffset=0  TranslationThetaOffsetUnits=deg  RotationMethod=None  RotationAngleUnits=deg  RotationStandardAxis=+Z  RotationAngle=0  RotationArbitraryAxis=[0 0 1]  FollAlignAxisA=+X  BaseAlignAxisA=+Y  FollAlignAxisB=+Y  BaseAlignAxisB=+Z  RotationSequenceAxes=FollowerAxes  RotationSequence=XYX  RotationSequenceAngles=[0 0 0]  RotationSequenceAnglesUnits=deg  RotationMatrix=[1 0 0; 0 1 0; 0 0 1]
  Transform2 : sm_lib/Frames and Transforms/Rigid Transform  TranslationMethod=Cartesian  TranslationStandardOffset=0  TranslationLengthUnit=in  TranslationStandardAxis=+Z  TranslationCartesianOffset=[-5.5118110236220464e-05 -0.085999999999999979 5.5118110236220464e-05]  TranslationROffset=0  TranslationROffsetUnits=m  TranslationZOffset=0  TranslationZOffsetUnits=m  TranslationThetaOffset=0  TranslationThetaOffsetUnits=deg  RotationMethod=ArbitraryAxis  RotationAngleUnits=rad  RotationStandardAxis=+Z  RotationAngle=1.5707963267948968  RotationArbitraryAxis=[-0 -0 -1]  FollAlignAxisA=+X  BaseAlignAxisA=+Y  FollAlignAxisB=+Y  BaseAlignAxisB=+Z  RotationSequenceAxes=FollowerAxes  RotationSequence=XYX  RotationSequenceAngles=[0 0 0]  RotationSequenceAnglesUnits=deg  RotationMatrix=[1 0 0; 0 1 0; 0 0 1]
  Transform3 : sm_lib/Frames and Transforms/Rigid Transform  TranslationMethod=Cartesian  TranslationStandardOffset=0  TranslationLengthUnit=in  TranslationStandardAxis=+Z  TranslationCartesianOffset=[-0.085999999999999979 5.5118110236220464e-05 5.5118110236220464e-05]  TranslationROffset=0  TranslationROffsetUnits=m  TranslationZOffset=0  TranslationZOffsetUnits=m  TranslationThetaOffset=0  TranslationThetaOffsetUnits=deg  RotationMethod=ArbitraryAxis  RotationAngleUnits=rad  RotationStandardAxis=+Z  RotationAngle=3.1415926535897931  RotationArbitraryAxis=[0 0 1]  FollAlignAxisA=+X  BaseAlignAxisA=+Y  FollAlignAxisB=+Y  BaseAlignAxisB=+Z  RotationSequenceAxes=FollowerAxes  RotationSequence=XYX  RotationSequenceAngles=[0 0 0]  RotationSequenceAnglesUnits=deg  RotationMatrix=[1 0 0; 0 1 0; 0 0 1]
  Transform4 : sm_lib/Frames and Transforms/Rigid Transform  TranslationMethod=Cartesian  TranslationStandardOffset=0  TranslationLengthUnit=in  TranslationStandardAxis=+Z  TranslationCartesianOffset=[5.5118110236220464e-05 0.085999999999999979 5.5118110236220464e-05]  TranslationROffset=0  TranslationROffsetUnits=m  TranslationZOffset=0  TranslationZOffsetUnits=m  TranslationThetaOffset=0  TranslationThetaOffsetUnits=deg  RotationMethod=ArbitraryAxis  RotationAngleUnits=rad  RotationStandardAxis=+Z  RotationAngle=1.5707963267948968  RotationArbitraryAxis=[0 0 1]  FollAlignAxisA=+X  BaseAlignAxisA=+Y  FollAlignAxisB=+Y  BaseAlignAxisB=+Z  RotationSequenceAxes=FollowerAxes  RotationSequence=XYX  RotationSequenceAngles=[0 0 0]  RotationSequenceAnglesUnits=deg  RotationMatrix=[1 0 0; 0 1 0; 0 0 1]
  Transform5 : sm_lib/Frames and Transforms/Rigid Transform  TranslationMethod=None  TranslationStandardOffset=0  TranslationLengthUnit=m  TranslationStandardAxis=+Z  TranslationCartesianOffset=[0 0 0]  TranslationROffset=0  TranslationROffsetUnits=m  TranslationZOffset=0  TranslationZOffsetUnits=m  TranslationThetaOffset=0  TranslationThetaOffsetUnits=deg  RotationMethod=None  RotationAngleUnits=deg  RotationStandardAxis=+Z  RotationAngle=0  RotationArbitraryAxis=[0 0 1]  FollAlignAxisA=+X  BaseAlignAxisA=+Y  FollAlignAxisB=+Y  BaseAlignAxisB=+Z  RotationSequenceAxes=FollowerAxes  RotationSequence=XYX  RotationSequenceAngles=[0 0 0]  RotationSequenceAnglesUnits=deg  RotationMatrix=[1 0 0; 0 1 0; 0 0 1]
  Motor Cmd 4 : PMIOPort  Side=Left
  Motor Cmd 3 : PMIOPort  Port=2  Side=Left
  Motor Cmd 2 : PMIOPort  Port=3  Side=Left
  Motor Cmd 1 : PMIOPort  Port=4  Side=Left
  w1 : PMIOPort  Port=5  Side=Left
  w2 : PMIOPort  Port=6  Side=Left
  w3 : PMIOPort  Port=7  Side=Left
  w4 : PMIOPort  Port=8  Side=Left
  ExtForce1 : PMIOPort  Port=9  Side=Right
  ExtForce2 : PMIOPort  Port=10  Side=Right
  ExtForce3 : PMIOPort  Port=11  Side=Right
  ExtForce4 : PMIOPort  Port=12  Side=Right
  6DoF : PMIOPort  Port=13  Side=Right
  connections:
  ExtForce2/RConn1 -- ASSY_ROTOR_END_3_RIGID/RConn2
  ExtForce4/RConn1 -- ASSY_ROTOR_END_1_RIGID/RConn2
  w1/RConn1 -- ASSY_ROTOR_END_1_RIGID/RConn1
  Motor Cmd 3/RConn1 -- ASSY_ROTOR_END_3_RIGID/LConn2
  w4/RConn1 -- ASSY_ROTOR_END_4_RIGID1/RConn1
  Motor Cmd 4/RConn1 -- ASSY_ROTOR_END_4_RIGID1/LConn2
  ExtForce1/RConn1 -- ASSY_ROTOR_END_4_RIGID1/RConn2
  ExtForce3/RConn1 -- ASSY_ROTOR_END_2_RIGID/RConn2
  w2/RConn1 -- ASSY_ROTOR_END_2_RIGID/RConn1
  Motor Cmd 2/RConn1 -- ASSY_ROTOR_END_2_RIGID/LConn2
  w3/RConn1 -- ASSY_ROTOR_END_3_RIGID/RConn1
  Motor Cmd 1/RConn1 -- ASSY_ROTOR_END_1_RIGID/LConn2
  HUB_1_RIGID/LConn1 -- Transform5/RConn1
  ASSY_ROTOR_END_3_RIGID/LConn1 -- Transform3/RConn1
  BOARD_1_RIGID/LConn1 -- Transform/RConn1
  ASSY_ROTOR_END_1_RIGID/LConn1 -- Transform1/RConn1
  Transform/LConn1 -- Transform4/LConn1 -- Transform5/LConn1 -- Transform3/LConn1 -- Transform2/LConn1 -- Transform1/LConn1 -- 6DoF/RConn1
  ASSY_ROTOR_END_2_RIGID/LConn1 -- Transform2/RConn1
  ASSY_ROTOR_END_4_RIGID1/LConn1 -- Transform4/RConn1

== system Quadrotor_Controller/Subsystem ==
  NavigationStates : Inport
  Enable_Control : Inport  Port=2
  Bus Selector1 : BusSelector  OutputSignals=VerticalVelocity,VerticalPosition
  Delay : Delay  DelayLength=1  InitialCondition=0  SampleTime=0.01
  Sum1 : Sum  Inputs=+|-
  Triggered Subsystem : Subsystem  TreatAsAtomicUnit=on
  Altitude_Rate : Outport
  Altitude_Ref : Outport  Port=2
  wires:
  Sum1/1 -> Altitude_Ref/1
  Enable_Control/1 -> Delay/1
  Delay/1 -> Triggered Subsystem/Trigger
  Bus Selector1/2 -> Sum1/1, Triggered Subsystem/1(In1)  "<VerticalPosition>"
  NavigationStates/1 -> Bus Selector1/1
  Bus Selector1/1 -> Altitude_Rate/1  "<VerticalVelocity>"
  Triggered Subsystem/1(Out1) -> Sum1/2

== system Quadrotor_Controller/Subsystem1 ==

== system Quadrotor_Controller/Subsystem2 ==

== system Quadrotor_Controller/Controller/FOPD ==
  note: FOPD controller
  In1 : Inport
  Fractional DD : Subsystem  mask{gam=0.9693, ww=[1e-4,1e4], n=6, kF1=on, kF=Oustaloup filter, Ts=0.01}
      mask prompts: gam "Derivative order gamma"; ww "Frequency range [wb,wh]"; n "Apprixmation order"; kF1 "Is a low-pass filter required?"; kF "Filter type"; Ts "Sampling period"
      mask init:
      | wb=ww(1); wh=ww(2); 
      | if kF==1, G=ousta_fod(gam,n,wb,wh);
      | else, G=new_fod(gam,n,wb,wh); end
      | %G=c2d(G,Ts,'tustin');
      | num=G.num{1}; den=G.den{1}; T=1/wh; str='Fractional\n';
      | if isnumeric(gam)
      | 	if gam>0, str=[str, 'Der  s^' num2str(gam) ];
      | 	else, str=[str, 'Int  s^{' num2str(gam) '}']; end
      | else, str=[str, 'Der  s^gam']; end
      | if kF1==1, G=G*tf(1,[T 1]); end
      mask TypeOptions kF: Oustaloup filter | Modified Oustaloup filter | Matsuda-Fujii filter
      mask Display: disp(str)
  Gain : Gain  Gain=7.9733
  Gain1 : Gain  Gain=0.2238
  Saturation1 : Saturate  UpperLimit=2e3  LowerLimit=-2e3
  Saturation2 : Saturate  UpperLimit=100  LowerLimit=-100
  Sum : Sum
  Out1 : Outport
  wires:
  Fractional DD/1(Out1) -> Saturation2/1  "DD_out"
  Gain1/1 -> Fractional DD/1(In1)  "DD_input"
  In1/1 -> Sum/1, Gain1/1  "P"
  Sum/1 -> Gain/1
  Gain/1 -> Saturation1/1
  Saturation1/1 -> Out1/1
  Saturation2/1 -> Sum/2  "D"

== system Quadrotor_Controller/Controller/FOPID ==
  note: FOPID controller
  In1 : Inport
  Fractional DD : Subsystem  mask{gam=0, ww=[1e-4,1e4], n=6, kF1=on, kF=Oustaloup filter, Ts=0.01}
      mask prompts: gam "Derivative order gamma"; ww "Frequency range [wb,wh]"; n "Apprixmation order"; kF1 "Is a low-pass filter required?"; kF "Filter type"; Ts "Sampling period"
      mask init: same as Quadrotor_Controller/Controller/FOPD/Fractional DD
      mask TypeOptions kF: Oustaloup filter | Modified Oustaloup filter | Matsuda-Fujii filter
      mask Display: disp(str)
  Fractional DD1 : Subsystem  mask{gam=1.5, ww=[1e-4,1e4], n=6, kF1=on, kF=Oustaloup filter, Ts=0.01}
      mask prompts: gam "Derivative order gamma"; ww "Frequency range [wb,wh]"; n "Apprixmation order"; kF1 "Is a low-pass filter required?"; kF "Filter type"; Ts "Sampling period"
      mask init: same as Quadrotor_Controller/Controller/FOPD/Fractional DD
      mask TypeOptions kF: Oustaloup filter | Modified Oustaloup filter | Matsuda-Fujii filter
      mask Display: disp(str)
  Gain1 : Gain  Gain=0
  Gain2 : Gain  Gain=2.6
  Gain3 : Gain  Gain=1.631
  Saturation1 : Saturate  UpperLimit=2e3  LowerLimit=-2e3
  Saturation2 : Saturate  UpperLimit=100  LowerLimit=-100
  Saturation3 : Saturate  UpperLimit=100  LowerLimit=-100
  Sum : Sum  Inputs=+++
  Out1 : Outport
  wires:
  Fractional DD/1(Out1) -> Saturation2/1  "DD_out"
  Gain1/1 -> Fractional DD/1(In1)  "DD_input"
  In1/1 -> Gain2/1, Gain3/1, Gain1/1  "P"
  Sum/1 -> Saturation1/1
  Saturation1/1 -> Out1/1
  Saturation2/1 -> Sum/2  "D"
  Gain2/1 -> Sum/1  "DD_input"
  Gain3/1 -> Fractional DD1/1(In1)  "DD_input"
  Fractional DD1/1(Out1) -> Saturation3/1  "DD_out"
  Saturation3/1 -> Sum/3  "D"

== system Quadrotor_Controller/Controller/FOPID NPM IRID with wrong plant ==
  note: FOPID controller
  In1 : Inport
  Discrete Transfer Fcn : DiscreteTransferFcn  Numerator=[1,-3.16336631308587,3.71959536925849,-1.96568707629962,0.436885459917815,-0.0273811687803932]  Denominator=[0.0935414346693485,-0.239486864955964,0.209356682991156,-0.0676440492684792,0.00352282535674651,0.000822432073709469]  SampleTime=0.01
  Discrete-Time Integrator : DiscreteIntegrator  SampleTime=0.01  ICPrevOutput=DiscIntNeverNeededParam  ICPrevScaledInput=DiscIntNeverNeededParam
  Gain2 : Gain  Gain=2.6
  Gain3 : Gain  Gain=1.631
  Saturation1 : Saturate  UpperLimit=2e3  LowerLimit=-2e3
  Saturation3 : Saturate  UpperLimit=100  LowerLimit=-100
  Sum : Sum  Inputs=+++
  Out1 : Outport
  wires:
  In1/1 -> Gain2/1, Gain3/1  "P"
  Sum/1 -> Saturation1/1
  Saturation1/1 -> Out1/1
  Gain2/1 -> Sum/1  "DD_input"
  Gain3/1 -> Discrete-Time Integrator/1  "DD_input"
  Discrete Transfer Fcn/1 -> Saturation3/1  "DD_out"
  Saturation3/1 -> Sum/3  "D"
  Discrete-Time Integrator/1 -> Discrete Transfer Fcn/1

== system Quadrotor_Controller/Controller/Tuned IOPID ==
  In1 : Inport
  Derivative : Derivative
  Discrete-Time Integrator : DiscreteIntegrator  SampleTime=-1  ICPrevOutput=DiscIntNeverNeededParam  ICPrevScaledInput=DiscIntNeverNeededParam
  Gain : Gain  Gain=10.7
  Gain1 : Gain  Gain=15.2
  Gain2 : Gain  Gain=1.66
  Gain3 : Gain
  Saturation : Saturate  UpperLimit=10  LowerLimit=-10
  Sum : Sum  Inputs=+++
  Sum1 : Sum  Inputs=-+|
  Sum2 : Sum  Inputs=|++
  Out1 : Outport
  wires:
  Sum/1 -> Sum1/1, Saturation/1
  Sum1/1 -> Gain3/1
  In1/1 -> Gain2/1, Gain/1, Gain1/1
  Sum2/1 -> Discrete-Time Integrator/1
  Derivative/1 -> Sum/3
  Gain/1 -> Sum/1
  Discrete-Time Integrator/1 -> Sum/2
  Gain1/1 -> Sum2/1
  Gain3/1 -> Sum2/2
  Gain2/1 -> Derivative/1
  Saturation/1 -> Sum1/2, Out1/1
